simulink model "Lab_2_WalecStozek"  (R2022b)
settings: Solver=VariableStepAuto  StartTime=0.0  StopTime=floor(20*Tmax)  RelTol=1e-3
values from neighbouring files (symbols this model uses):
  c1 = 3    [Lab_2.m]
  c2 = 1    [Lab_2.m]
  h1i = 0.2*h10    (= 0.0222222222222)    [Lab_2.m]
  H2 = 5    [Lab_2.m]
  h20 = (qwe/c2)^2    (= 1)    [Lab_2.m]
  h2i = 0.2*h20    (= 0.2)    [Lab_2.m]
  qdiff = 0.4    [Lab_2.m]
  qwe = 1    [Lab_2.m]
  R1 = 4    [Lab_2.m]
  R2 = 5    [Lab_2.m]
  Tmax = max(T1, T2)    [Lab_2.m]
undefined symbols (not defined in the file or in its folder): L, M
settings Model: Creator=Gabriel  LastModifiedBy=Gabriel
settings SolverCC: InitialStep=10^-6
settings DataIOCC: ReturnWorkspaceOutputs=off

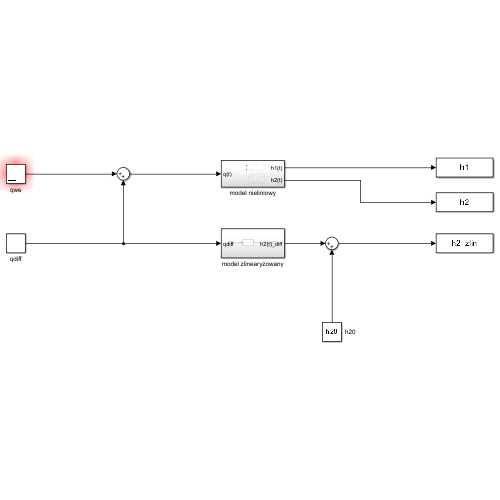
[thumbnail: Simulink's stored preview of the top-level diagram]
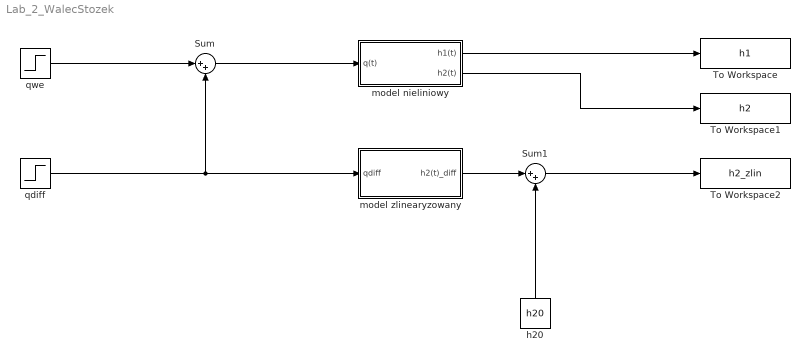
== system Lab_2_WalecStozek ==
  Sum : Sum  Inputs=|++
  Sum1 : Sum  Inputs=|++
  To Workspace : ToWorkspace  VariableName=h1  SaveFormat=Timeseries  SampleTime=10^-3
  To Workspace1 : ToWorkspace  VariableName=h2  SaveFormat=Timeseries  SampleTime=10^-3
  To Workspace2 : ToWorkspace  VariableName=h2_zlin  SaveFormat=Timeseries  SampleTime=10^-3
  h20 : Constant  Value=h20
  model nieliniowy : Subsystem
  model zlinearyzowany : Subsystem
  qdiff : Step  Time=floor(8*Tmax)  After=qdiff  SampleTime=0
  qwe : Step  Time=0  After=qwe  SampleTime=0
  wires:
  qwe/1 -> Sum/1
  Sum/1 -> model nieliniowy/1(q(t))
  qdiff/1 -> Sum/2, model zlinearyzowany/1(qdiff)
  model zlinearyzowany/1(h2(t)_diff) -> Sum1/1
  h20/1 -> Sum1/2
  Sum1/1 -> To Workspace2/1
  model nieliniowy/1(h1(t)) -> To Workspace/1
  model nieliniowy/2(h2(t)) -> To Workspace1/1

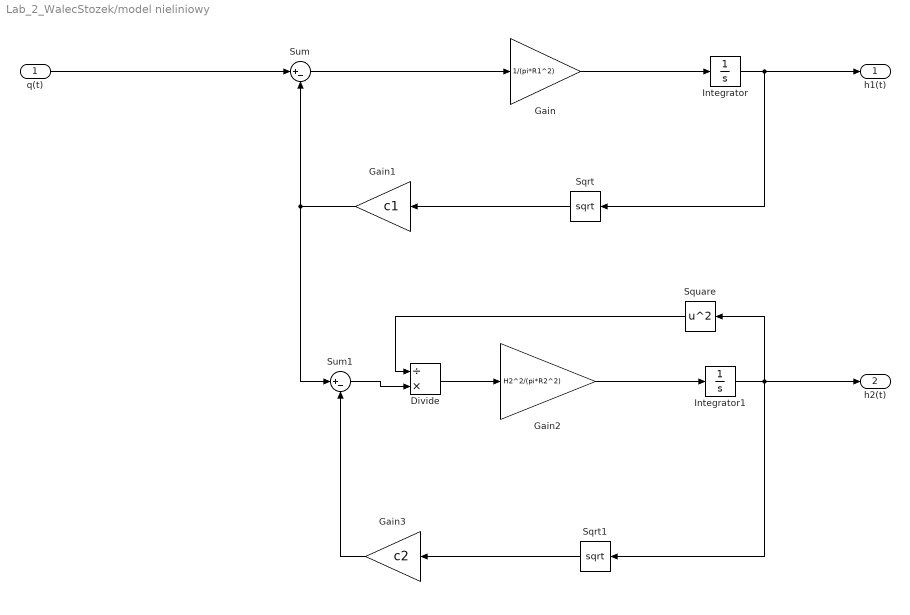
== system Lab_2_WalecStozek/model nieliniowy ==
  q(t) : Inport
  Divide : Product  Inputs=/*
  Gain : Gain  Gain=1/(pi*R1^2)
  Gain1 : Gain  Gain=c1
  Gain2 : Gain  Gain=H2^2/(pi*R2^2)
  Gain3 : Gain  Gain=c2
  Integrator : Integrator  InitialCondition=h1i
  Integrator1 : Integrator  InitialCondition=h2i
  Sqrt : Sqrt
  Sqrt1 : Sqrt
  Square : Math  Operator=square
  Sum : Sum  Inputs=|+-
  Sum1 : Sum  Inputs=|+-
  h1(t) : Outport
  h2(t) : Outport  Port=2
  wires:
  Gain1/1 -> Sum/2, Sum1/1
  Sum/1 -> Gain/1
  Sqrt/1 -> Gain1/1
  Integrator1/1 -> h2(t)/1, Square/1, Sqrt1/1
  Square/1 -> Divide/1
  Gain2/1 -> Integrator1/1
  Gain/1 -> Integrator/1
  Divide/1 -> Gain2/1
  Gain3/1 -> Sum1/2
  Sqrt1/1 -> Gain3/1
  Sum1/1 -> Divide/2
  q(t)/1 -> Sum/1
  Integrator/1 -> h1(t)/1, Sqrt/1

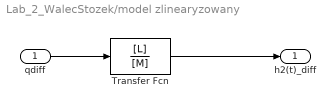
== system Lab_2_WalecStozek/model zlinearyzowany ==
  qdiff : Inport
  Transfer Fcn : TransferFcn  Numerator=[L]  Denominator=[M]
  h2(t)_diff : Outport
  wires:
  Transfer Fcn/1 -> h2(t)_diff/1
  qdiff/1 -> Transfer Fcn/1
